simulink model "W04_6_wrap"  (R2024b)
settings: Solver=ode4  StartTime=0.0  StopTime=60  FixedStep=0.05  RelTol=1e-3
values from neighbouring files (symbols this model uses):
  Kd_psi = 400    [W04_setup.m]
  Ki_psi = 0    [W04_setup.m]
  Kp_psi = 800    [W04_setup.m]
  N_max = 500    [W04_setup.m]
  psi0_deg = 0    [W04_setup.m]
  psi_wrap1_deg = 170    [W04_setup.m]
  psi_wrap2_deg = -170    [W04_setup.m]
  t_wrap1 = 5    [W04_setup.m]
  t_wrap2 = 20    [W04_setup.m]
  use_ssa = 1    [W04_setup.m]
settings Model: Creator=admin  LastModifiedBy=admin

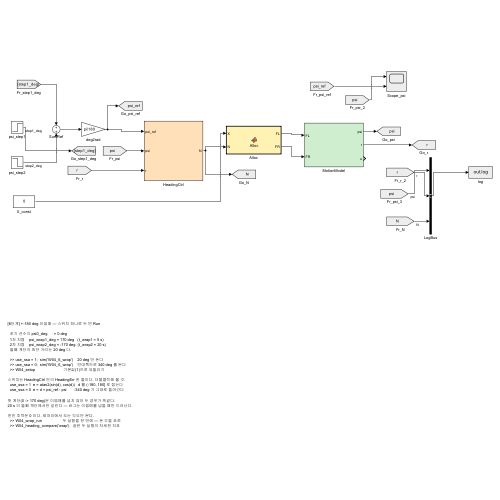
[thumbnail: Simulink's stored preview of the top-level diagram]
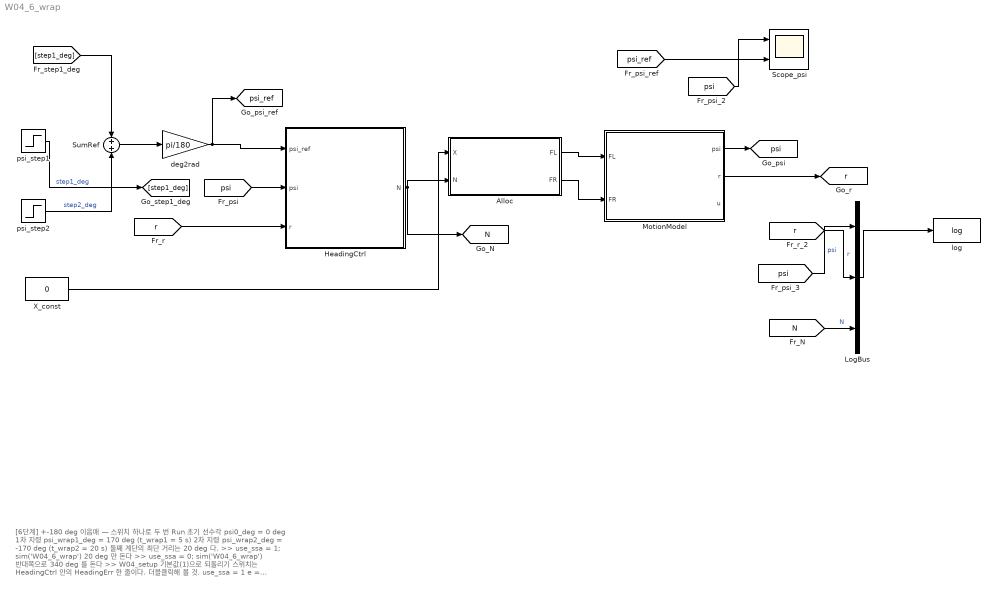
== system W04_6_wrap ==
  note: [6단계] +-180 deg 이음매 — 스위치 하나로 두 번 Run
      |
      |   초기 선수각 psi0_deg      = 0 deg
      |   1차 지령    psi_wrap1_deg = 170 deg   (t_wrap1 = 5 s)
      |   2차 지령    psi_wrap2_deg = -170 deg  (t_wrap2 = 20 s)
      |   둘째 계단의 최단 거리는 20 deg 다.
      |
      |   >> use_ssa = 1;  sim('W04_6_wrap')    20 deg 만 돈다
      |   >> use_ssa = 0;  sim('W04_6_wrap')    반대쪽으로 340 deg 를 돈다
      |   >> W04_setup                          기본값(1)으로 되돌리기
      |
      | 스위치는 HeadingCtrl 안의 HeadingErr 한 줄이다. 더블클릭해 볼 것.
      |   use_ssa = 1  e = atan2(sin(d), cos(d))   d 를 (-180, 180] 로 접는다
      |   use_ssa = 0  e = d = psi_ref - psi       -340 deg 가 그대로 들어간다
      |
      | 첫 계단(0 -> 170 deg)은 이음매를 넘지 않아 두 경우가 똑같다.
      | 20 s 의 둘째 계단에서만 갈린다 — 버그는 이음매를 넘을 때만 드러난다.
      |
      | 전진 추력은 0 이다. 제자리에서 도는 각도만 본다.
      |   >> W04_wrap_run                   두 실행을 한 번에 — 돈 각을 표로
      |   >> W04_heading_compare('wrap')   같은 두 실행의 자세한 지표
  Alloc : MATLAB Function  TreatAsAtomicUnit=on
  HeadingCtrl : Subsystem
  LogBus : BusCreator  Inputs=3
  MotionModel : Subsystem
  Scope_psi : Scope  NumInputPorts=2
  SumRef : Sum
  X_const : Constant  Value=0
  deg2rad : Gain  Gain=pi/180
  log : ToWorkspace  VariableName=log  SaveFormat=Timeseries  SampleTime=0.05
  psi_step1 : Step  Time=t_wrap1  After=psi_wrap1_deg  SampleTime=0
  psi_step2 : Step  Time=t_wrap2  After=psi_wrap2_deg - psi_wrap1_deg  SampleTime=0
  tag scope: N=global, psi=global, psi_ref=global, r=global
  wires:
  psi_step2/1 -> SumRef/2  "step2_deg"
  SumRef/1 -> deg2rad/1
  deg2rad/1 -> HeadingCtrl/1(psi_ref), [psi_ref]
  X_const/1 -> Alloc/1(X)
  Alloc/1(FL) -> MotionModel/1(FL)
  Alloc/2(FR) -> MotionModel/2(FR)
  MotionModel/1(psi) -> [psi]
  MotionModel/2(r) -> [r]
  [psi] -> HeadingCtrl/2(psi)
  [r] -> HeadingCtrl/3(r)
  [psi] -> Scope_psi/1
  [psi_ref] -> Scope_psi/2
  [r] -> LogBus/2  "r"
  [N] -> LogBus/3  "N"
  LogBus/1 -> log/1
  HeadingCtrl/1(N) -> Alloc/2(N), [N]
  psi_step1/1 -> [step1_deg]  "step1_deg"
  [step1_deg] -> SumRef/1
  [psi] -> LogBus/1  "psi"

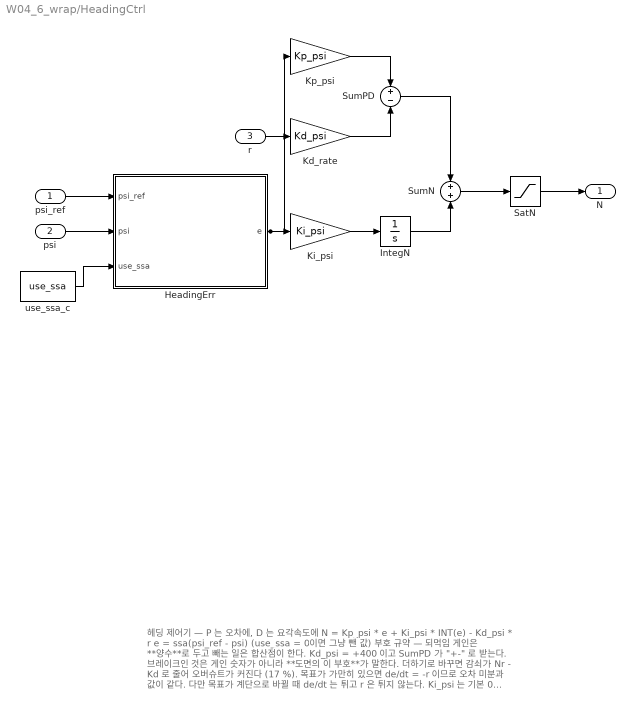
== system W04_6_wrap/HeadingCtrl ==
  note: 헤딩 제어기 — P 는 오차에, D 는 요각속도에
      |
      |     N = Kp_psi * e  +  Ki_psi * INT(e)  -  Kd_psi * r
      |     e = ssa(psi_ref - psi)   (use_ssa = 0 이면 그냥 뺀 값)
      |
      | 부호 규약 — 되먹임 게인은 **양수**로 두고 빼는 일은 합산점이 한다.
      | Kd_psi = +400 이고 SumPD 가 "+-" 로 받는다. 브레이크인 것은 게인
      | 숫자가 아니라 **도면의 이 부호**가 말한다.
      | 더하기로 바꾸면 감쇠가 Nr - Kd 로 줄어 오버슈트가 커진다 (17 %).
      |
      | 목표가 가만히 있으면 de/dt = -r 이므로 오차 미분과 값이 같다.
      | 다만 목표가 계단으로 바뀔 때 de/dt 는 튀고 r 은 튀지 않는다.
      |
      | Ki_psi 는 기본 0 이다. 한쪽 추진기가 약할 때(port_eff < 1)
      | PD 가 남기는 정상상태 오차를 없애는 자리다 (2-10 절 실습에서 켠다).
      | IntegN 은 **연속** 적분기이고 +-N_max 포화가 걸려 있다
      | (clamping 안티와인드업). 모델 솔버는 고정스텝 ode4 다.
      |
      | SatN 의 +-N_max = 500 N m 는 임의의 수가 아니다. 추진기만으로 낼 수
      | 있는 물리 한계가 2*b_half*F_max = 2*1.027135*250 = 513.57 N m 이고,
      | 500 은 그 97.4 % 다. 전진 추력 X 를 함께 쓰면 2*b_half*(F_max - X/2)
      | 로 줄어, X_head = 300 N 에서는 205.4 N m 가 진짜 한계다 (2-5 절 유도 5).
      |
      | 값은 전부 W04_setup.m — Kp_psi = 800, Kd_psi = +400.
      | 근거는 4주차 극배치 절과 W04_pole_place.m.
  psi_ref : Inport
  psi : Inport  Port=2
  r : Inport  Port=3
  HeadingErr : MATLAB Function  TreatAsAtomicUnit=on
  IntegN : Integrator  LimitOutput=on  UpperSaturationLimit=N_max  LowerSaturationLimit=-N_max
  Kd_rate : Gain  Gain=Kd_psi
  Ki_psi : Gain  Gain=Ki_psi
  Kp_psi : Gain  Gain=Kp_psi
  SatN : Saturate  UpperLimit=N_max  LowerLimit=-N_max
  SumN : Sum
  SumPD : Sum  Inputs=+-
  use_ssa_c : Constant  Value=use_ssa
  N : Outport
  wires:
  psi_ref/1 -> HeadingErr/1(psi_ref)
  psi/1 -> HeadingErr/2(psi)
  r/1 -> Kd_rate/1
  SumPD/1 -> SumN/1
  use_ssa_c/1 -> HeadingErr/3(use_ssa)
  Ki_psi/1 -> IntegN/1
  HeadingErr/1(e) -> Kp_psi/1, Ki_psi/1
  Kp_psi/1 -> SumPD/1
  IntegN/1 -> SumN/2
  Kd_rate/1 -> SumPD/2
  SumN/1 -> SatN/1
  SatN/1 -> N/1

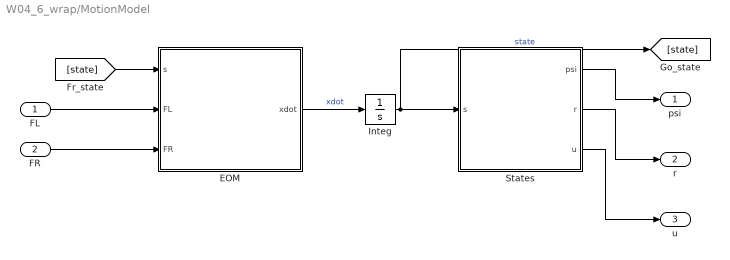
== system W04_6_wrap/MotionModel ==
  FL : Inport
  FR : Inport  Port=2
  EOM : MATLAB Function  TreatAsAtomicUnit=on
  Integ : Integrator  InitialCondition=[0;0;0;0;0;psi0_deg*pi/180]
  States : MATLAB Function  TreatAsAtomicUnit=on
  psi : Outport
  r : Outport  Port=2
  u : Outport  Port=3
  wires:
  FL/1 -> EOM/2(FL)
  FR/1 -> EOM/3(FR)
  EOM/1(xdot) -> Integ/1  "xdot"
  Integ/1 -> States/1(s), [state]  "state"
  States/1(psi) -> psi/1
  States/2(r) -> r/1
  States/3(u) -> u/1
  [state] -> EOM/1(s)

== matlab function W04_6_wrap/HeadingCtrl/HeadingErr ==
  data: psi_ref input; e output; psi input; use_ssa input
function e = HeadingErr(psi_ref, psi, use_ssa)
%#codegen
% Heading error [rad].
d = psi_ref - psi;
if use_ssa >= 0.5
    % ssa : shortest signed angle, wrapped to (-pi, pi]
    e = atan2(sin(d), cos(d));
else
    % no wrap : 170 deg -> -170 deg becomes -340 deg, not +20 deg
    e = d;
end

== matlab function W04_6_wrap/MotionModel/EOM ==
  data: s input; xdot output; FL input; FR input
function xdot = EOM(s, FL, FR)
%#codegen
% 3-DOF WAM-V equations of motion, NED (3주차 1-8 절).
%   s = [u v r x_n y_n psi]'
m = 211;  Izz = 653;  Xu = 100;  Xuu = 150;  Yv = 100;  Yvv = 100;
Nr = 800;  Nrr = 800;  b_half = 1.027135;
u = s(1); v = s(2); r = s(3); psi = s(6);
X = FL + FR;
N = (FL - FR)*b_half;
du = (X - (Xu + Xuu*abs(u))*u)/m + v*r;
dv = (  - (Yv + Yvv*abs(v))*v)/m - u*r;
dr = (N - (Nr + Nrr*abs(r))*r)/Izz;
xdot = [du; dv; dr;
        u*cos(psi) - v*sin(psi);
        u*sin(psi) + v*cos(psi);
        r];

== matlab function W04_6_wrap/MotionModel/States ==
  data: s input; psi output; r output; u output
function [psi, r, u] = States(s)
%#codegen
% Quat2Yaw 와 같은 출력 — 선수각은 [-pi, pi] 로 접는다
psi = atan2(sin(s(6)), cos(s(6)));
r = s(3);
u = s(1);

== matlab function W04_6_wrap/Alloc ==
  data: X input; FL output; N input; FR output
function [FL, FR] = Alloc(X, N)
%#codegen
% Differential thrust allocation for the 2-thruster WAM-V
%   X : surge force  [N]
%   N : yaw moment   [N*m], positive turns to starboard
B_half = 1.027135;      % half distance between thrusters [m]
Fmax   = 250;           % thrust limit per thruster [N]
FL = X/2 + N/(2*B_half);
FR = X/2 - N/(2*B_half);
FL = max(min(FL, Fmax), -Fmax);
FR = max(min(FR, Fmax), -Fmax);
